simulink model "Parcial_D"  (R2023b)
settings: Solver=ode8  StartTime=0.0  StopTime=30  FixedStep=Ts  RelTol=1e-3
values from neighbouring files (symbols this model uses):
  Ts = 4 / z    [Parcial.m]
  ue = sin(x1e)    [Parcial.m]
  x1e = deg2rad(150)    [Parcial.m]
  x2e = 0    [Parcial.m]
  ye = x1e    [Parcial.m]
libraries: cstblocks x1
settings Model: Creator=aghersin  LastModifiedBy=Usuario
settings SolverCC: AlgebraicLoopSolver=TrustRegion
settings DataIOCC: ReturnWorkspaceOutputs=off
settings OptimizationCC: LifeSpan=inf
settings DebuggingCC: UnconnectedInputMsg=warning  UnconnectedOutputMsg=warning  UnconnectedLineMsg=warning  SFExecutionAtInitializationDiag=none  ArithmeticOperatorsInVariantConditions=warning
settings ModelReferenceCC: EnableRefExpFcnMdlSchedulingChecks=on
settings SFSimCC: SimUseLocalCustomCode=off  CustomCodeUndefinedFunction=UseInterfaceOnly
settings RTWCC: RTWUseLocalCustomCode=off  DLArmComputeVersion=19.05
settings CodeAppCC: StateflowObjectComments=on

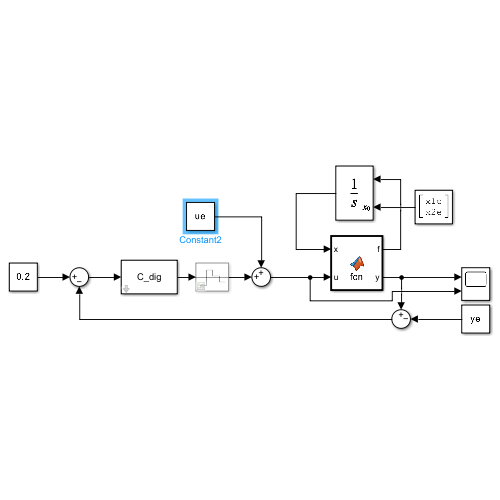
[thumbnail: Simulink's stored preview of the top-level diagram]
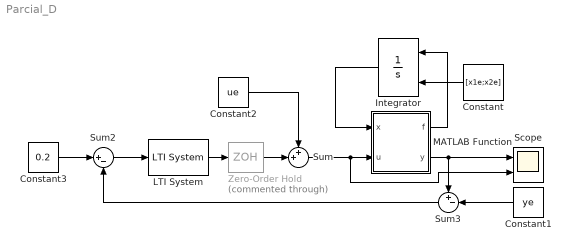
== system Parcial_D ==
  Constant : Constant  Value=[x1e;x2e]  VectorParams1D=off
  Constant1 : Constant  Value=ye
  Constant2 : Constant  Value=ue
  Constant3 : Constant  Value=0.2
  Integrator : Integrator  InitialConditionSource=external
  LTI System : cstblocks/LTI System  sys=C_dig  IC=[]  PadeOrder=0
  MATLAB Function : MATLAB Function  TreatAsAtomicUnit=on
  Scope : Scope  NumInputPorts=2
  Sum : Sum  Inputs=++|
  Sum2 : Sum  Inputs=|+-
  Sum3 : Sum  Inputs=+-|
  Zero-Order Hold : ZeroOrderHold  Commented=through  SampleTime=Ts
  wires:
  LTI System/1 -> Zero-Order Hold/1
  Constant2/1 -> Sum/1
  Sum2/1 -> LTI System/1
  MATLAB Function/1(f) -> Integrator/1
  Constant3/1 -> Sum2/1
  Sum3/1 -> Sum2/2
  Constant/1 -> Integrator/2
  MATLAB Function/2(y) -> Sum3/1, Scope/1
  Constant1/1 -> Sum3/2
  Zero-Order Hold/1 -> Sum/2
  Sum/1 -> Scope/2, MATLAB Function/2(u)
  Integrator/1 -> MATLAB Function/1(x)

== matlab function Parcial_D/MATLAB Function ==
  data: x input; u input; f output; y output
function [f,y] = fcn(x,u)

f1 = x(2);
f2 = u - sin(x(1));

f=[f1; f2];

y=x(1);
